simulink model "project3_sim"  (R2023b)
settings: Solver=VariableStepAuto  StartTime=0.0  StopTime=0.05  RelTol=1e-3
values from neighbouring files (symbols this model uses):
  frequency = 1500    [project3.m]
undefined symbols (not defined in the file or in its folder): denc, denp, numc, nump
settings Model: Creator=trinc  LastModifiedBy=trinc

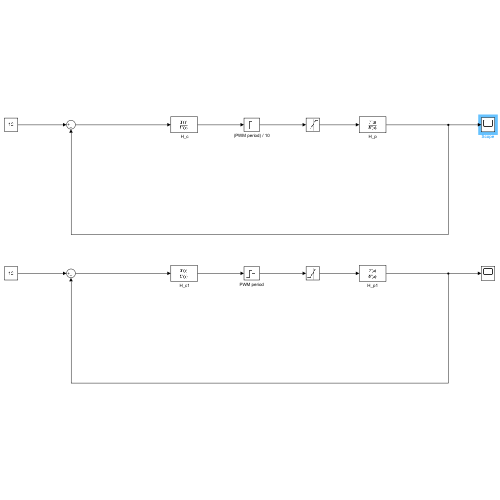
[thumbnail: Simulink's stored preview of the top-level diagram]
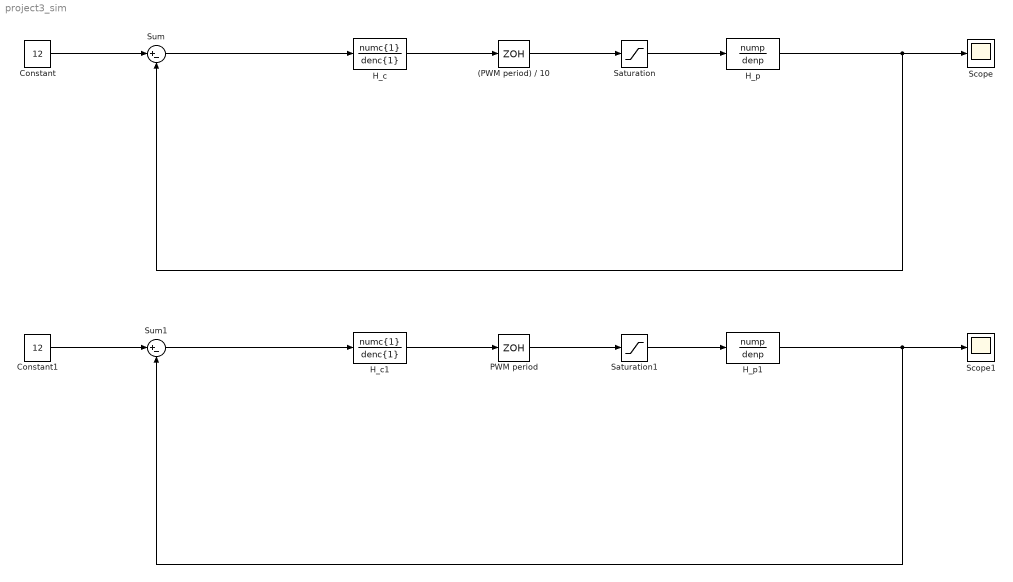
== system project3_sim ==
  " H_c" : TransferFcn  Numerator=numc{1}  Denominator=denc{1}
  " H_c1" : TransferFcn  Numerator=numc{1}  Denominator=denc{1}
  (PWM period) / 10 : ZeroOrderHold  SampleTime=1/frequency/10
  Constant : Constant  Value=12
  Constant1 : Constant  Value=12
  H_p : TransferFcn  Numerator=nump  Denominator=denp
  H_p1 : TransferFcn  Numerator=nump  Denominator=denp
  PWM period : ZeroOrderHold  SampleTime=1/frequency
  Saturation : Saturate  UpperLimit=1  LowerLimit=0
  Saturation1 : Saturate  UpperLimit=1  LowerLimit=0
  Scope : Scope
  Scope1 : Scope
  Sum : Sum  Inputs=|+-
  Sum1 : Sum  Inputs=|+-
  wires:
  Sum/1 -> " H_c"/1
  " H_c"/1 -> (PWM period) / 10/1
  (PWM period) / 10/1 -> Saturation/1
  Saturation/1 -> H_p/1
  H_p/1 -> Sum/2, Scope/1
  Constant/1 -> Sum/1
  Constant1/1 -> Sum1/1
  H_p1/1 -> Sum1/2, Scope1/1
  PWM period/1 -> Saturation1/1
  Saturation1/1 -> H_p1/1
  " H_c1"/1 -> PWM period/1
  Sum1/1 -> " H_c1"/1
